simulink model "CurrPowerLimCalc"  (R2023b)
settings: Solver=FixedStepDiscrete  StartTime=0.0  StopTime=40000  RelTol=1e-3  EnableMultiTasking=on
undefined symbols (not defined in the file or in its folder): M, M0, Ns, OverCellVoltageLimit, Q, R, R0, ts, UnderCellVoltageLimit
settings Model: DataDictionary=DD_CurrPowerLimCalc.sldd  EnableAccessToBaseWorkspace=off  ExtModeTrigDuration=5  Creator=cpatel  LastModifiedBy=Alkhouly
settings SolverCC: AlgebraicLoopSolver=TrustRegion  AutoInsertRateTranBlk=on
settings DataIOCC: ExternalInput=Battery  SaveOutput=off  SaveTime=off  SignalLoggingName=logsOut
settings OptimizationCC: DefaultParameterBehavior=Inlined  UseDivisionForNetSlopeComputation=on  UseFloatMulNetSlope=on  DefaultUnderspecifiedDataType=single  UseSpecifiedMinMax=on  PassReuseOutputArgsAs=Individual arguments  ZeroExternalMemoryAtStartup=off  ZeroInternalMemoryAtStartup=off  NoFixptDivByZeroProtection=on  EfficientFloat2IntCast=on  LifeSpan=inf  MaxStackSize=64  OptimizeBlockOrder=speed  DifferentSizesBufferReuse=on  EfficientTunableParamExpr=on
settings DebuggingCC: SignalInfNanChecking=error  SaveWithParameterizedLinksMsg=none  CheckExecutionContextPreStartOutputMsg=on  IntegerOverflowMsg=error  ParameterPrecisionLossMsg=none  ParameterTunabilityLossMsg=error  UnconnectedInputMsg=warning  UnconnectedOutputMsg=warning  UnconnectedLineMsg=warning  AssertControl=DisableAll  PregeneratedLibrarySubsystemCodeDiagnostic=none  SFUnexpectedBacktrackingDiag=warning  SFNoUnconditionalDefaultTransitionDiag=warning  SFExecutionAtInitializationDiag=none  ArithmeticOperatorsInVariantConditions=warning
settings HardwareCC: ProdBitPerPointer=32  ProdBitPerSizeT=32  ProdBitPerPtrDiffT=32  ProdLargestAtomicInteger=Long  ProdLargestAtomicFloat=Double  ProdEndianess=BigEndian  ProdWordSize=32  ProdHWDeviceType=Texas Instruments->TMS570 Cortex-R4
settings ModelReferenceCC: EnableRefExpFcnMdlSchedulingChecks=on  ModelReferenceNumInstancesAllowed=Single  PropagateSignalLabelsOutOfModel=off
settings SFSimCC: SimUseLocalCustomCode=off  MATLABDynamicMemAlloc=off  CustomCodeUndefinedFunction=UseInterfaceOnly
settings RTWCC: Description=Embedded Coder  SystemTargetFile=ert.tlc  GenCodeOnly=on  TemplateMakefile=ert_default_tmf  GenerateReport=on  RTWUseLocalCustomCode=off  Toolchain=TI ARM Code Generation Tools | gmake  IncludeHyperlinkInReport=on  GenerateTraceInfo=on  GenerateTraceReport=on  GenerateTraceReportSl=on  GenerateTraceReportSf=on  GenerateTraceReportEml=on  GenerateWebview=on  GenerateCodeMetricsReport=on
settings CodeAppCC: ForceParamTrailComments=on  IgnoreCustomStorageClasses=off  MaxIdLength=51  OperatorAnnotations=on  SimulinkDataObjDesc=on  SFDataObjDesc=on  MangleLength=4  InsertBlockDesc=on  ReqsInCode=on
settings ERTTargetCC: UtilityFuncGeneration=Shared location  IncludeMdlTerminateFcn=off  CombineSignalStateStructs=on  SuppressErrorStatus=on  SupportNonFinite=off  SupportComplex=off  ParenthesesLevel=Maximum  CastingMode=Standards  GenerateSharedConstants=off  ERTCustomFileTemplate=example_file_process.tlc  PreserveExpressionOrder=on  PreserveIfCondition=on  EnableSignedLeftShifts=off  EnableSignedRightShifts=off
settings ConfigComp: CovMetricSettings=dcw  CovSaveCumulativeToWorkspaceVar=on  CovSaveSingleToWorkspaceVar=on  CovExternalEMLEnable=off  CovSFcnEnable=off  DVMode=DesignErrorDetection  DVMaxProcessTime=7000  DVTestSuiteOptimization=Auto  DVDetectDeadLogic=on  DVDetectIntegerOverflow=off

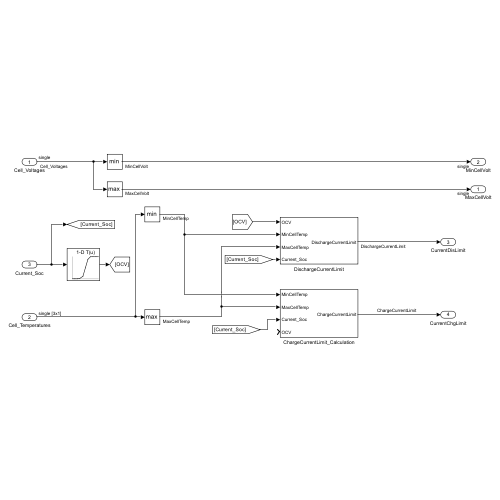
[thumbnail: Simulink's stored preview of the top-level diagram]
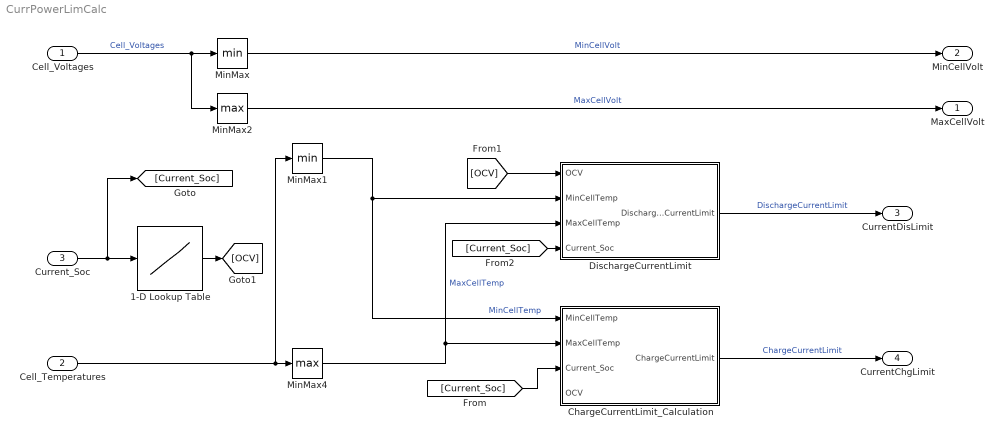
== system CurrPowerLimCalc ==
  Cell_Voltages : Inport  OutDataTypeStr=single  PortDimensions=Ns*1  SampleTime=[0.10000000000000001,0]
  Cell_Temperatures : Inport  Port=2  OutDataTypeStr=single  PortDimensions=[3 1]  SampleTime=[0.10000000000000001,0]
  Current_Soc : Inport  Port=3
  1-D Lookup Table : Lookup_n-D  NumberOfTableDimensions=1  BreakpointsForDimension1=[-5:5]  Table=tanh([-5:5])  InternalRulePriority=Speed  RndMeth=Simplest
  ChargeCurrentLimit_Calculation : Subsystem
  DischargeCurrentLimit : Subsystem
  MinMax : MinMax
  MinMax1 : MinMax
  MinMax2 : MinMax  Function=max
  MinMax4 : MinMax  Function=max
  MaxCellVolt : Outport  OutDataTypeStr=single  PortDimensions=1  SampleTime=[0.10000000000000001,0]  VectorParamsAs1DForOutWhenUnconnected=off
  MinCellVolt : Outport  Port=2  OutDataTypeStr=single  PortDimensions=1  SampleTime=[0.10000000000000001,0]  VectorParamsAs1DForOutWhenUnconnected=off
  CurrentDisLimit : Outport  Port=3
  CurrentChgLimit : Outport  Port=4
  wires:
  ChargeCurrentLimit_Calculation/1(ChargeCurrentLimit) -> CurrentChgLimit/1  "ChargeCurrentLimit"
  DischargeCurrentLimit/1(DischargeCurrentLimit) -> CurrentDisLimit/1  "DischargeCurrentLimit"
  Cell_Voltages/1 -> MinMax2/1, MinMax/1  "Cell_Voltages"
  Cell_Temperatures/1 -> MinMax1/1, MinMax4/1
  MinMax2/1 -> MaxCellVolt/1  "MaxCellVolt"
  MinMax/1 -> MinCellVolt/1  "MinCellVolt"
  MinMax4/1 -> DischargeCurrentLimit/3(MaxCellTemp), ChargeCurrentLimit_Calculation/2(MaxCellTemp)  "MaxCellTemp"
  MinMax1/1 -> DischargeCurrentLimit/2(MinCellTemp), ChargeCurrentLimit_Calculation/1(MinCellTemp)  "MinCellTemp"
  [Current_Soc] -> ChargeCurrentLimit_Calculation/3(Current_Soc)
  Current_Soc/1 -> 1-D Lookup Table/1, [Current_Soc]
  1-D Lookup Table/1 -> [OCV]
  [OCV] -> DischargeCurrentLimit/1(OCV)
  [Current_Soc] -> DischargeCurrentLimit/4(Current_Soc)

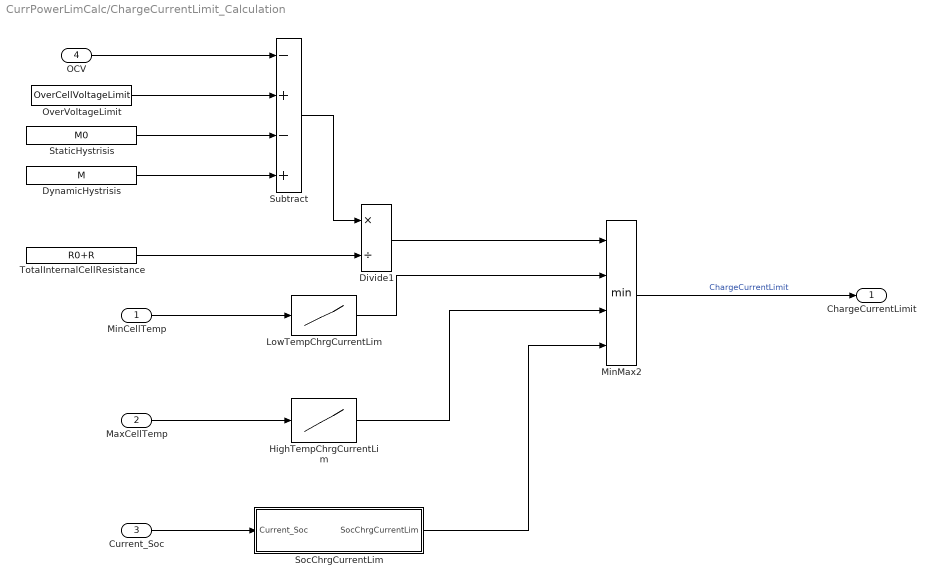
== system CurrPowerLimCalc/ChargeCurrentLimit_Calculation ==
  MinCellTemp : Inport
  MaxCellTemp : Inport  Port=2
  Current_Soc : Inport  Port=3
  OCV : Inport  Port=4
  Divide1 : Product  Inputs=*/
  DynamicHystrisis : Constant  Value=M  OutDataTypeStr=single  SampleTime=ts
  HighTempChrgCurrentLim : Lookup_n-D  NumberOfTableDimensions=1  BreakpointsForDimension1=273.15+[-30:1:70]  Table=50*(1-tanh(273.15+[-30:1:70]-273.15-50))/2  InternalRulePriority=Speed  RndMeth=Simplest
  LowTempChrgCurrentLim : Lookup_n-D  NumberOfTableDimensions=1  BreakpointsForDimension1=273.15+[-30:1:70]  Table=50*(1+tanh(273.15+[-30:1:70]-(273.15)))/2  InternalRulePriority=Speed  RndMeth=Simplest
  MinMax2 : MinMax  Inputs=4
  OverVoltageLimit : Constant  Value=OverCellVoltageLimit  OutDataTypeStr=single  SampleTime=ts
  SocChrgCurrentLim : Subsystem  InitFcn=Q=40
  StaticHystrisis : Constant  Value=M0  OutDataTypeStr=single  SampleTime=ts
  Subtract : Sum  Inputs=-+-+
  TotalInternalCellResistance : Constant  Value=R0+R  OutDataTypeStr=single  SampleTime=ts
  ChargeCurrentLimit : Outport  VectorParamsAs1DForOutWhenUnconnected=off
  wires:
  Divide1/1 -> MinMax2/1
  TotalInternalCellResistance/1 -> Divide1/2
  MinCellTemp/1 -> LowTempChrgCurrentLim/1
  MaxCellTemp/1 -> HighTempChrgCurrentLim/1
  HighTempChrgCurrentLim/1 -> MinMax2/3
  LowTempChrgCurrentLim/1 -> MinMax2/2
  Current_Soc/1 -> SocChrgCurrentLim/1(Current_Soc)
  SocChrgCurrentLim/1(SocChrgCurrentLim) -> MinMax2/4
  OverVoltageLimit/1 -> Subtract/2
  OCV/1 -> Subtract/1
  Subtract/1 -> Divide1/1
  StaticHystrisis/1 -> Subtract/3
  DynamicHystrisis/1 -> Subtract/4
  MinMax2/1 -> ChargeCurrentLimit/1  "ChargeCurrentLimit"

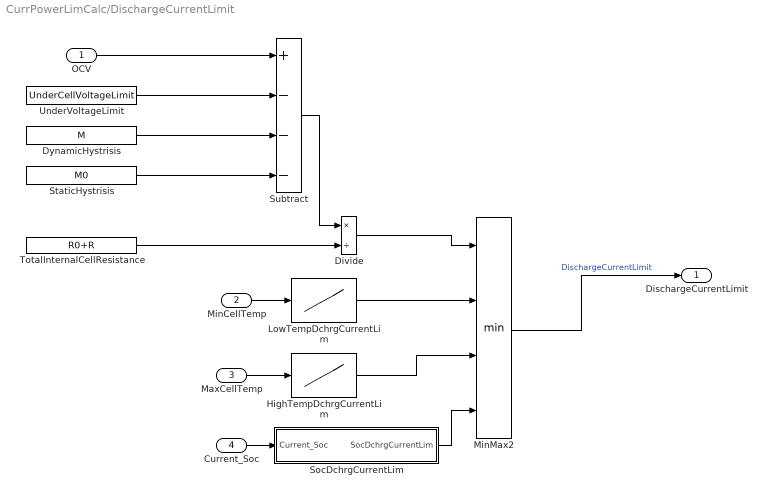
== system CurrPowerLimCalc/DischargeCurrentLimit ==
  OCV : Inport
  MinCellTemp : Inport  Port=2
  MaxCellTemp : Inport  Port=3
  Current_Soc : Inport  Port=4
  Divide : Product  Inputs=*/
  DynamicHystrisis : Constant  Value=M  OutDataTypeStr=single  SampleTime=ts
  HighTempDchrgCurrentLim : Lookup_n-D  NumberOfTableDimensions=1  BreakpointsForDimension1=273.15+[-30:1:70]  Table=100*(1-tanh(273.15+[-30:1:70]-273.15-50))/2  InternalRulePriority=Speed  RndMeth=Simplest
  LowTempDchrgCurrentLim : Lookup_n-D  NumberOfTableDimensions=1  BreakpointsForDimension1=273.15+[-30:1:70]  Table=100*(1+tanh(273.15+[-30:1:70]-(273.15)))/2  InternalRulePriority=Speed  RndMeth=Simplest
  MinMax2 : MinMax  Inputs=4
  SocDchrgCurrentLim : Subsystem  InitFcn=Q=40
  StaticHystrisis : Constant  Value=M0  OutDataTypeStr=single  SampleTime=ts
  Subtract : Sum  Inputs=+---
  TotalInternalCellResistance : Constant  Value=R0+R  OutDataTypeStr=single  SampleTime=ts
  UnderVoltageLimit : Constant  Value=UnderCellVoltageLimit  OutDataTypeStr=single  SampleTime=ts
  DischargeCurrentLimit : Outport  VectorParamsAs1DForOutWhenUnconnected=off
  wires:
  MinMax2/1 -> DischargeCurrentLimit/1  "DischargeCurrentLimit"
  Divide/1 -> MinMax2/1
  OCV/1 -> Subtract/1
  TotalInternalCellResistance/1 -> Divide/2
  Subtract/1 -> Divide/1
  UnderVoltageLimit/1 -> Subtract/2
  MaxCellTemp/1 -> HighTempDchrgCurrentLim/1
  MinCellTemp/1 -> LowTempDchrgCurrentLim/1
  HighTempDchrgCurrentLim/1 -> MinMax2/3
  LowTempDchrgCurrentLim/1 -> MinMax2/2
  Current_Soc/1 -> SocDchrgCurrentLim/1(Current_Soc)
  SocDchrgCurrentLim/1(SocDchrgCurrentLim) -> MinMax2/4
  DynamicHystrisis/1 -> Subtract/3
  StaticHystrisis/1 -> Subtract/4

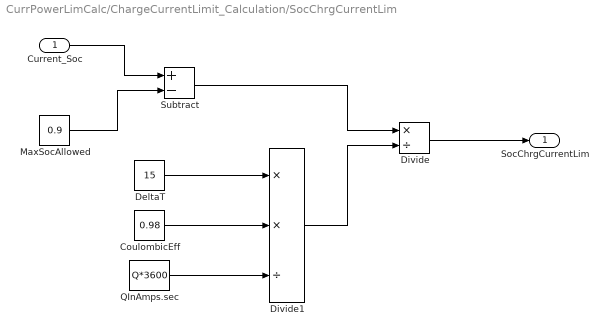
== system CurrPowerLimCalc/ChargeCurrentLimit_Calculation/SocChrgCurrentLim ==
  Current_Soc : Inport
  CoulombicEff : Constant  Value=0.98
  DeltaT : Constant  Value=15
  Divide : Product  Inputs=*/
  Divide1 : Product  Inputs=**/
  MaxSocAllowed : Constant  Value=0.9
  QInAmps.sec : Constant  Value=Q*3600
  Subtract : Sum  Inputs=+-
  SocChrgCurrentLim : Outport
  wires:
  Divide/1 -> SocChrgCurrentLim/1
  Current_Soc/1 -> Subtract/1
  MaxSocAllowed/1 -> Subtract/2
  Subtract/1 -> Divide/1
  Divide1/1 -> Divide/2
  DeltaT/1 -> Divide1/1
  CoulombicEff/1 -> Divide1/2
  QInAmps.sec/1 -> Divide1/3

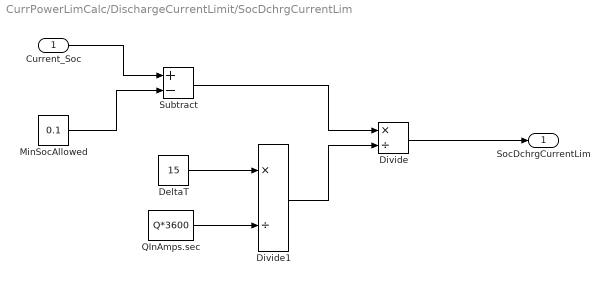
== system CurrPowerLimCalc/DischargeCurrentLimit/SocDchrgCurrentLim ==
  Current_Soc : Inport
  DeltaT : Constant  Value=15
  Divide : Product  Inputs=*/
  Divide1 : Product  Inputs=*/
  MinSocAllowed : Constant  Value=0.1
  QInAmps.sec : Constant  Value=Q*3600
  Subtract : Sum  Inputs=+-
  SocDchrgCurrentLim : Outport
  wires:
  Current_Soc/1 -> Subtract/1
  MinSocAllowed/1 -> Subtract/2
  Subtract/1 -> Divide/1
  DeltaT/1 -> Divide1/1
  QInAmps.sec/1 -> Divide1/2
  Divide1/1 -> Divide/2
  Divide/1 -> SocDchrgCurrentLim/1
